simulink subsystem "OL_PTI"  (R2025a)
settings: Solver=VariableStepAuto  StartTime=0.0  StopTime=10.0  RelTol=1e-3
undefined symbols (not defined in the file): FC
libraries: simulink x2
settings Model: Creator=gurt1  LastModifiedBy=17036
settings RTWCC: GPUComputeCapability=3.5

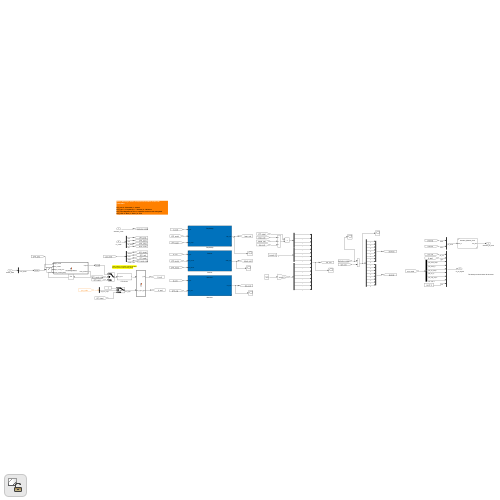
[thumbnail: Simulink's stored preview of the top-level diagram]
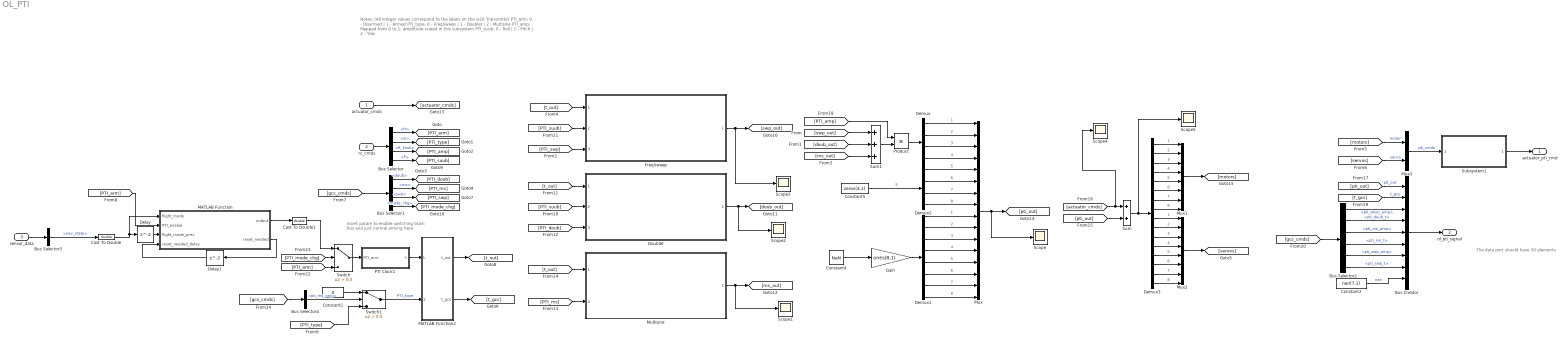
== system OL_PTI ==
  note: insert param to enable switching btwn this and just normal arming here
  note: Notes: (All integer values correspond to the labels on the ix20 Transmitter
      |
      | PTI_arm: 0 - Disarmed | 1 - Armed
      | PTI_type: 0 - FreqSweep | 1 - Doublet | 2 - Multisine
      | PTI_amp: Mapped from 0 to 1, amplitude scaled in this subsystem
      | PTI_suub: 0 - Roll | 1 - Pitch | 2 - Yaw
  note: The data port should have 30 elements
  actuator_cmds : Inport
  rc_cmds : Inport  Port=2
  sensor_data : Inport  Port=3
  Bus Creator : BusCreator  Inputs=9
  Bus Selector : BusSelector  OutputSignals=switches.H,switches.G,switches.R_knob,switches.F
  Bus Selector1 : BusSelector  OutputSignals=PTI.PTI.doub,PTI.PTI.ms,PTI.PTI.swp,PTI.PTI.mode_chg
  Bus Selector2 : BusSelector  OutputSignals=PTI.PTI.doub.pti_doub_amp,PTI.PTI.doub.pti_doub_t,PTI.PTI.ms.pti_ms_amp,PTI.PTI.ms.pti_ms_t,PTI.PTI.swp.pti_swp_amp,PTI.PTI.swp.pti_swp_t
  Bus Selector3 : BusSelector  OutputSignals=nav_state
  Bus Selector4 : BusSelector  OutputSignals=PTI.PTI.ms.pti_ms_only
  Cast To Double : DataTypeConversion  OutDataTypeStr=double  SaturateOnIntegerOverflow=off  RndMeth=Floor
  Cast To Double1 : DataTypeConversion  OutDataTypeStr=double  SaturateOnIntegerOverflow=off  RndMeth=Floor
  Constant1 : Constant  Value=0
  Constant2 : Constant  Value=nan(7,1)
  Constant4 : Constant  Value=NaN
  Constant5 : Constant  Value=zeros(4,1)
  Delay : Delay
  Delay1 : Delay
  Demux : Demux
  Demux1 : Demux  Outputs=8
  Demux2 : Demux
  Demux3 : Demux  Outputs=16
  Doublet : Subsystem  ReferencedSubsystem=Doublet
  FreqSweep : Subsystem  ReferencedSubsystem=FreqSweep
  Gain : Gain  Gain=ones(8,1)
  MATLAB Function : MATLAB Function  TreatAsAtomicUnit=on
  MATLAB Function2 : MATLAB Function  TreatAsAtomicUnit=on
  Multisine : Subsystem  ReferencedSubsystem=Multisine
  Mux : Mux  Inputs=16
  Mux1 : Mux  Inputs=8
  Mux2 : Mux  Inputs=8
  Mux3 : Mux  Inputs=2
  PTI Clock1 : Subsystem
  Product : Product
  Scope{,1..5} (6 alike) : Scope
      Scope1 settings: DataLoggingVariableName=ScopeData2
      Scope2 settings: DataLoggingVariableName=ScopeData3
      Scope3 settings: DataLoggingVariableName=ScopeData4
      Scope4 settings: DataLoggingVariableName=ScopeData5
  Subsystem1 : Subsystem  ReferencedSubsystem=Actuator_Manual_Cmd
  Sum : Sum
  Sum1 : Sum  Inputs=+++
  Switch : Switch  Criteria=u2 > Threshold  Threshold=0.5  SaturateOnIntegerOverflow=off  InputSameDT=off
  Switch1 : Switch  Criteria=u2 > Threshold  Threshold=0.5  SaturateOnIntegerOverflow=off  InputSameDT=off
  actuator_pti_cmd : Outport
  ol_pti_signal : Outport  Port=2
  wires:
  [PTI_mode_chg] -> Switch/2
  Bus Selector1/4 -> [PTI_mode_chg]  "<mode_chg>"
  Switch/1 -> PTI Clock1/1(PTI_arm)
  [PTI_arm] -> Switch/3
  Subsystem1/1 -> actuator_pti_cmd/1
  [PTI_suub] -> FreqSweep/2
  Bus Selector2/6 -> Bus Creator/8  "<pti_swp_t>"
  Bus Selector2/5 -> Bus Creator/7  "<pti_swp_amp>"
  Bus Selector2/4 -> Bus Creator/6  "<pti_ms_t>"
  Bus Selector2/3 -> Bus Creator/5  "<pti_ms_amp>"
  Bus Selector2/2 -> Bus Creator/4  "<pti_doub_t>"
  Bus Selector2/1 -> Bus Creator/3  "<pti_doub_amp>"
  [gcs_cmds] -> Bus Selector2/1
  [t_gcs] -> Bus Creator/2  "t_gcs"
  Constant2/1 -> Bus Creator/9  "nan"
  MATLAB Function2/2(t_gcs) -> [t_gcs]
  [PTI_amp] -> Product/1
  Sum1/1 -> Product/2
  Product/1 -> Demux/1
  [pti_out] -> Bus Creator/1  "pti_out"
  Mux2/1 -> [servos]
  Mux1/1 -> [motors]
  Demux3/11 -> Mux2/3  "3"
  Demux3/10 -> Mux2/2  "2"
  Demux3/9 -> Mux2/1  "1"
  Demux3/16 -> Mux2/8  "8"
  Demux3/13 -> Mux2/5  "5"
  Demux3/15 -> Mux2/7  "7"
  Demux3/14 -> Mux2/6  "6"
  Demux3/8 -> Mux1/8  "8"
  Demux3/7 -> Mux1/7  "7"
  Demux3/6 -> Mux1/6  "6"
  Demux3/5 -> Mux1/5  "5"
  Demux3/4 -> Mux1/4  "4"
  Demux3/3 -> Mux1/3  "3"
  Demux3/2 -> Mux1/2  "2"
  Demux3/1 -> Mux1/1  "1"
  Sum/1 -> Scope5/1, Demux3/1
  Demux1/4 -> Mux/12  "4"
  Demux1/3 -> Mux/11  "3"
  Demux1/8 -> Mux/16  "8"
  Demux1/2 -> Mux/10  "2"
  Constant4/1 -> Gain/1
  Demux1/1 -> Mux/9  "1"
  Demux1/6 -> Mux/14  "6"
  Gain/1 -> Demux1/1
  Demux1/5 -> Mux/13  "5"
  Demux1/7 -> Mux/15  "7"
  [actuator_cmds] -> Scope4/1, Sum/1
  [pti_out] -> Sum/2
  Mux/1 -> Scope/1, [pti_out]
  actuator_cmds/1 -> [actuator_cmds]
  [ms_out] -> Sum1/3
  [doub_out] -> Sum1/2
  [swp_out] -> Sum1/1
  FreqSweep/1 -> Scope3/1, [swp_out]
  Multisine/1 -> Scope1/1, [ms_out]
  Doublet/1 -> Scope2/1, [doub_out]
  [PTI_ms] -> Multisine/2
  [t_out] -> Multisine/1
  [PTI_suub] -> Doublet/2
  Bus Selector/4 -> [PTI_suub]  "<F>"
  [t_out] -> Doublet/1
  [PTI_doub] -> Doublet/3
  [t_out] -> FreqSweep/1
  MATLAB Function2/1(t_out) -> [t_out]
  PTI Clock1/1(t) -> MATLAB Function2/1(t)
  Cast To Double1/1 -> Switch/1
  [PTI_swp] -> FreqSweep/3
  Bus Selector1/2 -> [PTI_ms]  "<ms>"
  Bus Selector1/1 -> [PTI_doub]  "<doub>"
  Bus Selector1/3 -> [PTI_swp]  "<swp>"
  Bus Selector/3 -> [PTI_amp]  "<R_knob>"
  Bus Selector/2 -> [PTI_type]  "<G>"
  rc_cmds/1 -> Bus Selector/1
  Bus Creator/1 -> ol_pti_signal/1
  Demux/1 -> Mux/1  "1"
  Demux/4 -> Mux/4  "4"
  Demux2/2 -> Mux/6  "6"
  Demux2/3 -> Mux/7  "7"
  Demux2/4 -> Mux/8  "8"
  Demux/3 -> Mux/3  "3"
  Demux/2 -> Mux/2  "2"
  Demux2/1 -> Mux/5  "5"
  Constant5/1 -> Demux2/1  "5"
  [motors] -> Mux3/1  "motor"
  [servos] -> Mux3/2  "servo"
  Mux3/1 -> Subsystem1/1  "pti_cmds"
  [gcs_cmds] -> Bus Selector1/1
  Demux3/12 -> Mux2/4  "4"
  Bus Selector/1 -> [PTI_arm]  "<H>"
  Cast To Double/1 -> MATLAB Function/1(flight_mode), Delay/1
  Delay/1 -> MATLAB Function/3(flight_mode_prev)
  [PTI_arm] -> MATLAB Function/2(PTI_enable)
  MATLAB Function/2(reset_needed) -> Delay1/1
  Delay1/1 -> MATLAB Function/4(reset_needed_delay)
  MATLAB Function/1(output) -> Cast To Double1/1
  Bus Selector4/1 -> Switch1/2  "<pti_ms_only>"
  [gcs_cmds] -> Bus Selector4/1
  Constant1/1 -> Switch1/1
  [PTI_type] -> Switch1/3
  Switch1/1 -> MATLAB Function2/2(PTI_type)  "PTI_type"
  sensor_data/1 -> Bus Selector3/1
  Bus Selector3/1 -> Cast To Double/1  "<nav_state>"

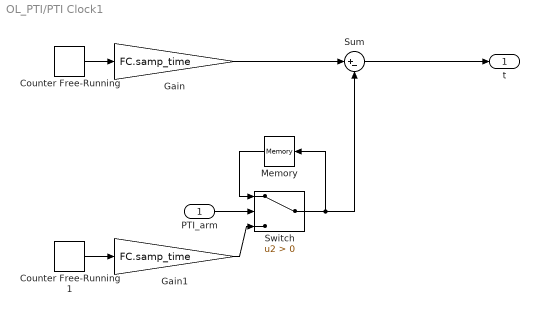
== system OL_PTI/PTI Clock1 ==
  PTI_arm : Inport
  Counter Free-Running : simulink/Sources/Counter Free-Running  NumBits=32  tsamp=-1
  Counter Free-Running1 : simulink/Sources/Counter Free-Running  NumBits=32  tsamp=-1
  Gain : Gain  Gain=FC.samp_time  OutDataTypeStr=double
  Gain1 : Gain  Gain=FC.samp_time  OutDataTypeStr=double
  Memory : Memory
  Sum : Sum  Inputs=|+-
  Switch : Switch  Criteria=u2 > Threshold  SaturateOnIntegerOverflow=off  InputSameDT=off
  t : Outport
  wires:
  Counter Free-Running/1 -> Gain/1
  Gain/1 -> Sum/1
  Counter Free-Running1/1 -> Gain1/1
  Gain1/1 -> Switch/3
  Switch/1 -> Sum/2, Memory/1
  Memory/1 -> Switch/1
  PTI_arm/1 -> Switch/2
  Sum/1 -> t/1

== matlab function OL_PTI/MATLAB Function2 ==
  data: t input; t_out output; PTI_type input; t_gcs output
function [t_out,t_gcs] = fcn(t, PTI_type)

t_gcs = t;

if PTI_type == 0
    t_out = [t,0,0];
elseif PTI_type == 1
    t_out = [0,t,0];
elseif PTI_type == 2
    t_out = [0,0,t];
else
    t_out = [0,0,0];
end

== matlab function OL_PTI/MATLAB Function ==
  data: flight_mode input; output output; PTI_enable input; flight_mode_prev input; reset_needed_delay input; reset_needed output
function [output,reset_needed] = checkFlightMode(flight_mode, PTI_enable, flight_mode_prev, reset_needed_delay)
    % Output true (1) if flight_mode has not changed since PTI_enable was enabled
    
    % Initialize output
    output = 0;
    reset_needed = 0;

    % Take care of reset_needed if applicable
    if reset_needed_delay == 1
        if PTI_enable == 1
            reset_needed = 1;
            output = 0;
            return
        end
    end
    
    % Check if PTI_enable is off
    if PTI_enable == 1
        output = 1;
    end

    % Check if PTI_enable is on and flight_mode has changed
    if flight_mode ~= flight_mode_prev && reset_needed == 0
        output = 0;
        reset_needed = 1;
    end
end
